simulink model "simulink_L2"  (R2018a)
settings: Solver=FixedStepDiscrete  StartTime=0.0  StopTime=10.0  RelTol=1e-3
settings Model: Creator=Labit  LastModifiedBy=vladi

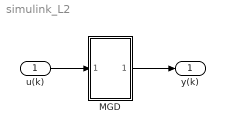
== system simulink_L2 ==
  u(k) : Inport
  "MGD " : Subsystem
  y(k) : Outport
  wires:
  "MGD "/1(y(k)) -> y(k)/1
  u(k)/1 -> "MGD "/1(u(k))

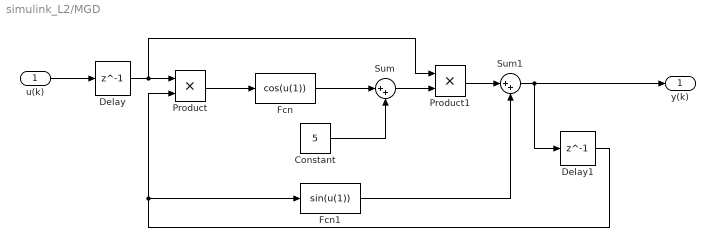
== system simulink_L2/MGD  ==
  u(k) : Inport
  Constant : Constant  Value=5
  Delay : Delay  DelayLength=1  InitialCondition=0
  Delay1 : Delay  DelayLength=1  InitialCondition=0
  Fcn : Fcn  Expr=cos(u(1))
  Fcn1 : Fcn  Expr=sin(u(1))
  Product : Product
  Product1 : Product
  Sum : Sum  Inputs=|++
  Sum1 : Sum  Inputs=|++
  y(k) : Outport
  wires:
  Delay/1 -> Product1/1, Product/1
  Delay1/1 -> Fcn1/1, Product/2
  Product1/1 -> Sum1/1
  Fcn/1 -> Sum/1
  Fcn1/1 -> Sum1/2
  Sum1/1 -> y(k)/1, Delay1/1
  Sum/1 -> Product1/2
  Product/1 -> Fcn/1
  Constant/1 -> Sum/2
  u(k)/1 -> Delay/1
